simulink model "cstr_ampc_ctrl"  (R2020a)
settings: Solver=ode45  StartTime=0  StopTime=200  MaxStep=0.5*Ts  RelTol=1e-3  EnableMultiTasking=on
values from neighbouring files (symbols this model uses):
  Ts = 0.1    [A.m]
undefined symbols (not defined in the file or in its folder): CA0, R, u0, x0
libraries: mympclib x2, simulink x1, simulink_extras x1
settings Model: Creator=The MathWorks, Inc.  LastModifiedBy=kohei
settings DataIOCC: ExternalInput=ExtIn  InitialState=[311.267; 8.5695]  SaveFormat=Structure  SaveOutput=off  SaveTime=off  ReturnWorkspaceOutputs=off  SignalLoggingName=logsOut
settings OptimizationCC: BooleanDataType=off  DefaultParameterBehavior=Inlined  InlineInvariantSignals=on  BufferReuse=off  ExpressionDepthLimit=2147483647  InitFltsAndDblsToZero=on  LifeSpan=inf
settings DebuggingCC: SaveWithParameterizedLinksMsg=none  UnderspecifiedInitializationDetection=Classic  MergeDetectMultiDrivingBlocksExec=none  CheckExecutionContextPreStartOutputMsg=on  CheckExecutionContextRuntimeOutputMsg=on  SignalResolutionControl=TryResolveAllWithWarning  MultiTaskDSMMsg=warning  MultiTaskCondExecSysMsg=none  StateNameClashWarn=warning  SFUnexpectedBacktrackingDiag=warning  SFNoUnconditionalDefaultTransitionDiag=warning  SFExecutionAtInitializationDiag=none  ArithmeticOperatorsInVariantConditions=warning
settings HardwareCC: ProdBitPerPointer=32  ProdBitPerSizeT=32  ProdBitPerPtrDiffT=32  ProdLargestAtomicFloat=None  ProdIntDivRoundTo=Undefined  ProdEndianess=Unspecified  ProdWordSize=32  ProdHWDeviceType=32-bit Generic  TargetBitPerPointer=64  TargetBitPerSizeT=64  TargetBitPerPtrDiffT=64  TargetLongLongMode=on  TargetIntDivRoundTo=Zero  TargetEndianess=LittleEndian  TargetWordSize=64  TargetHWDeviceType=MATLAB Host  ProdEqTarget=off
settings ModelReferenceCC: PropagateSignalLabelsOutOfModel=off
settings SFSimCC: SimUseLocalCustomCode=off  CustomCodeUndefinedFunction=UseInterfaceOnly
settings RTWCC: RTWUseLocalCustomCode=off
settings CodeAppCC: StateflowObjectComments=on
settings GRTTargetCC: TargetFcnLib=ansi_tfl_tmw.mat  TargetLangStandard=C89/C90 (ANSI)  CombineOutputUpdateFcns=off  GRTInterface=on
settings ConfigComp: CovMetricSettings=dw  CovHtmlReporting=on  CovSaveCumulativeToWorkspaceVar=on  CovSaveSingleToWorkspaceVar=on  CovExternalEMLEnable=off  CovSFcnEnable=off

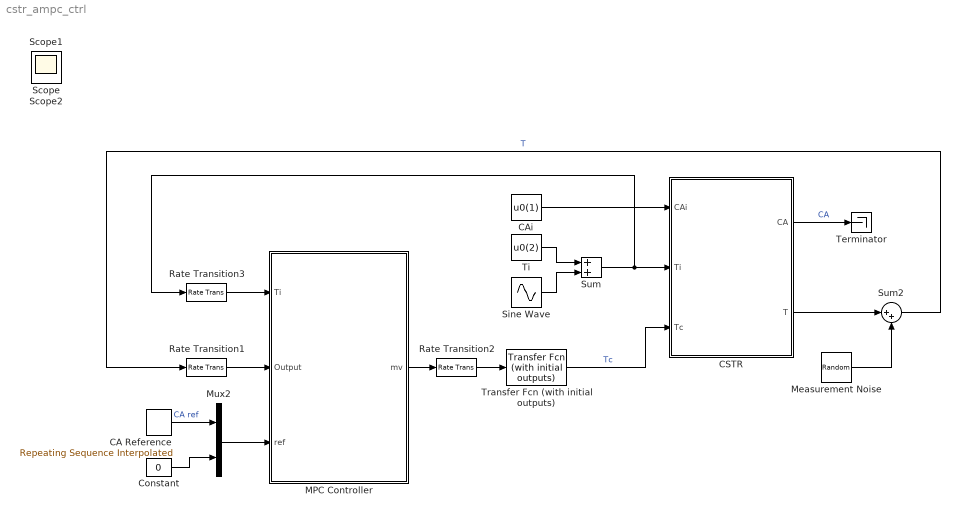
== system cstr_ampc_ctrl ==
  CA Reference : simulink/Sources/Repeating Sequence Interpolated  OutValues=[CA0,CA0, 2, 2]  TimeValues="[0 50  150 200]"  LookUpMeth=Interpolation-Use End Values  tsamp=Ts  OutMin=[]  OutMax=[]  OutDataTypeStr=double  OutputDataTypeScalingMode=double  OutDataType=fixdt(0,8)  OutScaling=2^-10
  CAi : Constant  Value=u0(1)
  CSTR : Subsystem
  Constant : Constant  Value=0  SampleTime=Ts
  MPC Controller : Subsystem  TreatAsAtomicUnit=on
  Measurement Noise : RandomNumber  SampleTime=Ts
  Mux2 : Mux  Inputs=2
  Rate Transition1 : RateTransition  InitialCondition=x0(2)
  Rate Transition2 : RateTransition  InitialCondition=u0(3)
  Rate Transition3 : RateTransition  InitialCondition=u0(2)
  Sine Wave : Sin  Frequency=0.1  SampleTime=0
  Sum : Sum
  Sum2 : Sum  Inputs=|++
  Terminator : Terminator
  Ti : Constant  Value=u0(2)
  Transfer Fcn (with initial outputs) : simulink_extras/Additional Linear/Transfer Fcn (with initial outputs)  N=[1]  D="[1  1]"  Y0=u0(3)  U0=u0(3)
  Scope : Scope
  Scope1 : Scope
  Scope2 : Scope
  wires:
  CAi/1 -> CSTR/1(CAi)
  Ti/1 -> Sum/1
  Sine Wave/1 -> Sum/2
  CSTR/2(T) -> Sum2/1
  CSTR/1(CA) -> Terminator/1  "CA"
  Measurement Noise/1 -> Sum2/2
  MPC Controller/1(mv) -> Rate Transition2/1
  Sum/1 -> Rate Transition3/1, CSTR/2(Ti)
  CA Reference/1 -> Mux2/1  "CA ref"
  Constant/1 -> Mux2/2
  Rate Transition3/1 -> MPC Controller/1(Ti)
  Rate Transition1/1 -> MPC Controller/2(Output)
  Mux2/1 -> MPC Controller/3(ref)
  Transfer Fcn (with initial outputs)/1 -> CSTR/3(Tc)  "Tc"
  Rate Transition2/1 -> Transfer Fcn (with initial outputs)/1
  Sum2/1 -> Rate Transition1/1  "T"

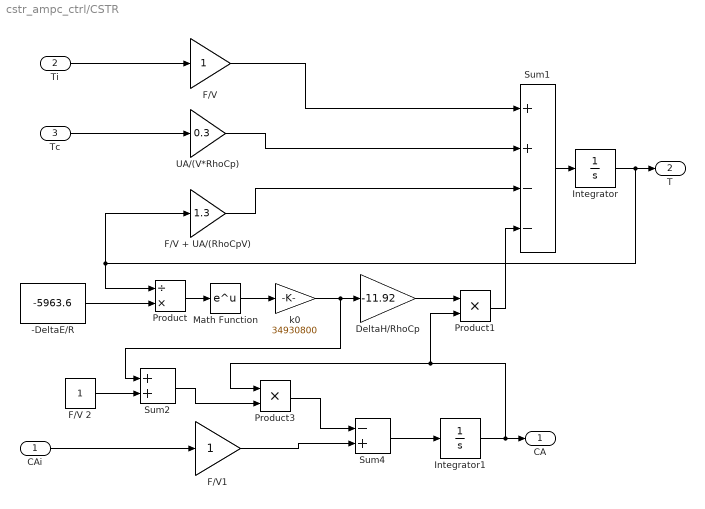
== system cstr_ampc_ctrl/CSTR ==
  CAi : Inport
  Ti : Inport  Port=2
  Tc : Inport  Port=3
  -DeltaE/R : Constant  Value=-5963.6
  DeltaH/RhoCp : Gain  Gain=-11.92  SaturateOnIntegerOverflow=on  OutDataTypeStr=Inherit: Same as input  ParamDataTypeStr=Inherit: Same as input
  F/V : Gain  SaturateOnIntegerOverflow=on  OutDataTypeStr=Inherit: Same as input  ParamDataTypeStr=Inherit: Same as input
  F/V + UA/(RhoCpV) : Gain  Gain=1.3  SaturateOnIntegerOverflow=on  OutDataTypeStr=Inherit: Same as input  ParamDataTypeStr=Inherit: Same as input
  F/V 2 : Constant
  F/V1 : Gain  SaturateOnIntegerOverflow=on  OutDataTypeStr=Inherit: Same as input  ParamDataTypeStr=Inherit: Same as input
  Integrator : Integrator  InitialCondition=x0(2)  LimitOutput=on  LowerSaturationLimit=0
  Integrator1 : Integrator  InitialCondition=x0(1)  LimitOutput=on  LowerSaturationLimit=0
  Math Function : Math  SignedPower=on  SaturateOnIntegerOverflow=on
  Product : Product  Inputs=/*  InputSameDT=on  RndMeth=Zero  SaturateOnIntegerOverflow=on  OutDataTypeStr=Inherit: Same as first input
  Product1 : Product  InputSameDT=on  RndMeth=Zero  SaturateOnIntegerOverflow=on  OutDataTypeStr=Inherit: Same as first input
  Product3 : Product  InputSameDT=on  RndMeth=Zero  SaturateOnIntegerOverflow=on  OutDataTypeStr=Inherit: Same as first input
  Sum1 : Sum  Inputs=++--  InputSameDT=on  SaturateOnIntegerOverflow=on  OutDataTypeStr=Inherit: Same as first input
  Sum2 : Sum  InputSameDT=on  SaturateOnIntegerOverflow=on  OutDataTypeStr=Inherit: Same as first input
  Sum4 : Sum  Inputs=-+  InputSameDT=on  SaturateOnIntegerOverflow=on  OutDataTypeStr=Inherit: Same as first input
  UA/(V*RhoCp) : Gain  Gain=0.3  SaturateOnIntegerOverflow=on  OutDataTypeStr=Inherit: Same as input  ParamDataTypeStr=Inherit: Same as input
  k0 : Gain  Gain=34930800  SaturateOnIntegerOverflow=on  OutDataTypeStr=Inherit: Same as input  ParamDataTypeStr=Inherit: Same as input
  CA : Outport
  T : Outport  Port=2
  wires:
  Sum2/1 -> Product3/2
  Tc/1 -> UA/(V*RhoCp)/1
  CAi/1 -> F/V1/1
  Ti/1 -> F/V/1
  F/V1/1 -> Sum4/2
  F/V 2/1 -> Sum2/2
  Integrator1/1 -> CA/1, Product3/1, Product1/2
  Sum4/1 -> Integrator1/1
  Product3/1 -> Sum4/1
  -DeltaE/R/1 -> Product/2
  k0/1 -> Sum2/1, DeltaH/RhoCp/1
  Product1/1 -> Sum1/4
  DeltaH/RhoCp/1 -> Product1/1
  Math Function/1 -> k0/1
  Product/1 -> Math Function/1
  F/V + UA/(RhoCpV)/1 -> Sum1/3
  UA/(V*RhoCp)/1 -> Sum1/2
  Integrator/1 -> T/1, F/V + UA/(RhoCpV)/1, Product/1
  Sum1/1 -> Integrator/1
  F/V/1 -> Sum1/1

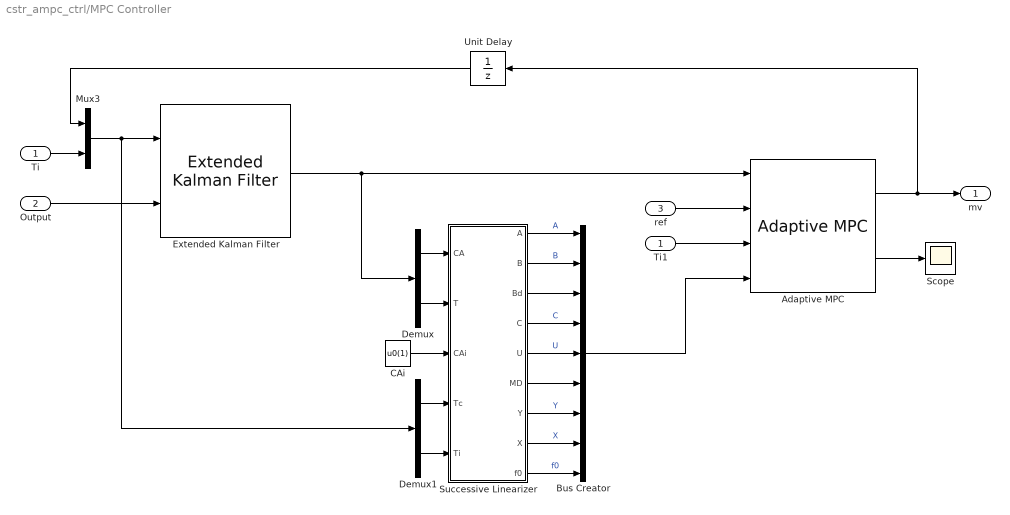
== system cstr_ampc_ctrl/MPC Controller ==
  Ti : Inport
  Output : Inport  Port=2
  ref : Inport  Port=3
  Adaptive MPC : mympclib/Adaptive MPC  params=params  numState=2  numRef=2  numMV=1  Ts=Ts  enableDist=on  numDist=1  enableSlack=off  enableStatus=on  enableMVseq=off
      settings: SourceProductName=My MPC Library
  Bus Creator : BusCreator  Inputs=9  OutDataTypeStr=Bus: sysBus
  CAi : Constant  Value=u0(1)
  Demux : Demux  Outputs=2
  Demux1 : Demux  Outputs=2
  Extended Kalman Filter : mympclib/Extended Kalman Filter  stateFunction='f'  jacobianStateFunction='A'  measurementFunction='h'  jacobianMeasurmentFunction='C'  Bv=Bv  Q=Q  R=R  xhat0=xhat0  P0=P0  Ts=Ts  numState=2  numOutput=1  enableP=off  enableG=off
      settings: SourceProductName=My MPC Library
  Mux3 : Mux  Inputs=2
  Scope : Scope
  Successive Linearizer : MATLAB Function  TreatAsAtomicUnit=on  SystemSampleTime=Ts
  Ti1 : InportShadow
  Unit Delay : UnitDelay  InitialCondition=u0(3)  SampleTime=-1  HasFrameUpgradeWarning=on
  mv : Outport
  wires:
  Successive Linearizer/5(U) -> Bus Creator/5  "U"
  Successive Linearizer/9(f0) -> Bus Creator/9  "f0"
  Bus Creator/1 -> Adaptive MPC/4
  Successive Linearizer/1(A) -> Bus Creator/1  "A"
  Successive Linearizer/7(Y) -> Bus Creator/7  "Y"
  Successive Linearizer/8(X) -> Bus Creator/8  "X"
  Successive Linearizer/6(MD) -> Bus Creator/6
  Successive Linearizer/3(Bd) -> Bus Creator/3
  Successive Linearizer/4(C) -> Bus Creator/4  "C"
  Adaptive MPC/1 -> mv/1, Unit Delay/1
  Successive Linearizer/2(B) -> Bus Creator/2  "B"
  Demux/1 -> Successive Linearizer/1(CA)
  Demux/2 -> Successive Linearizer/2(T)
  CAi/1 -> Successive Linearizer/3(CAi)
  Mux3/1 -> Demux1/1, Extended Kalman Filter/1
  Unit Delay/1 -> Mux3/1
  Demux1/2 -> Successive Linearizer/5(Ti)
  Demux1/1 -> Successive Linearizer/4(Tc)
  ref/1 -> Adaptive MPC/2
  Output/1 -> Extended Kalman Filter/2
  Ti/1 -> Mux3/2
  Extended Kalman Filter/1 -> Adaptive MPC/1, Demux/1
  Ti1/1 -> Adaptive MPC/3
  Adaptive MPC/2 -> Scope/1

== matlab function cstr_ampc_ctrl/MPC Controller/Successive Linearizer ==
  data: CA input; A output; T input; B output; Bd output; CAi input; Tc input; Ti input; C output; U output; MD output; Y output; X output; f0 output; Ts parameter
function [A,B,Bd,C,U,MD,Y,X,f0] = fcn(CA,T,CAi,Tc,Ti,Ts)
[A,B,Bd,C,U,MD,Y,X,f0] = calcSuccessiveLinear(T,CA,CAi,Ti,Tc,Ts);
